simulink model "Mixer_TestBed_org"  (Simulink 10.0)
settings: Solver=FixedStepDiscrete  StartTime=0.0  StopTime=1  FixedStep=1  RelTol=1e-3  EnableMultiTasking=on
undefined symbols (not defined in the file): MWS, stripchar_TMATS
libraries: Lib_Turbo_Mixer_TMATS x1
settings Model: Creator=jwchapm2  LastModifiedBy=annonymous
settings DataIOCC: LimitDataPoints=on
settings OptimizationCC: ExpressionDepthLimit=2147483647
settings DebuggingCC: SolverPrmCheckMsg=warning  StateNameClashWarn=warning
settings GRTTargetCC: GeneratePreprocessorConditionals=Disable all  CombineOutputUpdateFcns=on  GRTInterface=off
settings ConfigComp: CovExternalEMLEnable=off

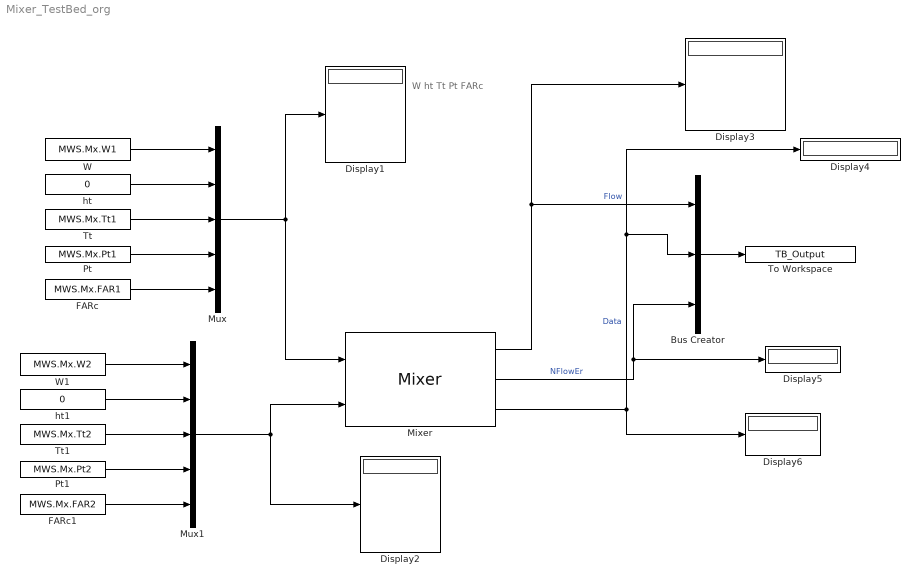
== system Mixer_TestBed_org ==
  note: W
      | ht
      | Tt
      | Pt
      | FARc
  Bus Creator : BusCreator  Inputs=3
  Display{1..6} (6 alike) : Display
  FARc : Constant  Value=MWS.Mx.FAR1
  FARc1 : Constant  Value=MWS.Mx.FAR2
  Mixer : Lib_Turbo_Mixer_TMATS/Mixer  Aphy1_M=MWS.Mx.A1  Aphy2_M=MWS.Mx.A2  s_M_Imp1_M=MWS.Mx.I1  s_M_Imp2_M=MWS.Mx.I2  s_M_V1_M=MWS.Mx.V1  s_M_V2_M=MWS.Mx.V2  Y_M_FARVec_M=[0; 0.0050; 0.0100; 0.0150; 0.0200; 0.0250; 0.0300]  T_M_RtArray_M="[0.0686;    0.0686;    0.0686;    0.0686;    0.0686;    0.0686;    0.0686]"  X_M_TVec_M=[300 10000]  T_M_gammaArray_M=[ 1.4 1.4 1.4 1.4 1.4 1.4 1.4; 1.4 1.4 1.4 1.4 1.4 1.4 1.4]  iDesign_M=2  SWPS_M=0  BPRDes_M=0.5  MNDes_M=0.4  FVar_M=strcat('iDes_',stripchar_TMATS(gcb),'.bin')
  Mux : Mux  Inputs=5
  Mux1 : Mux  Inputs=5
  Pt : Constant  Value=MWS.Mx.Pt1
  Pt1 : Constant  Value=MWS.Mx.Pt2
  To Workspace : ToWorkspace  VariableName=TB_Output  SampleTime=-1
  Tt : Constant  Value=MWS.Mx.Tt1
  Tt1 : Constant  Value=MWS.Mx.Tt2
  W : Constant  Value=MWS.Mx.W1
  W1 : Constant  Value=MWS.Mx.W2
  ht : Constant  Value=0
  ht1 : Constant  Value=0
  wires:
  W/1 -> Mux/1
  FARc/1 -> Mux/5
  Tt/1 -> Mux/3
  Pt/1 -> Mux/4
  Mux/1 -> Mixer/1, Display1/1
  Mixer/1 -> Display3/1, Bus Creator/1  "Flow"
  Mixer/3 -> Bus Creator/2, Display4/1, Display6/1  "Data"
  Mixer/2 -> Bus Creator/3, Display5/1  "NFlowEr"
  Bus Creator/1 -> To Workspace/1
  ht/1 -> Mux/2
  Mux1/1 -> Mixer/2, Display2/1
  W1/1 -> Mux1/1
  FARc1/1 -> Mux1/5
  Tt1/1 -> Mux1/3
  Pt1/1 -> Mux1/4
  ht1/1 -> Mux1/2
